simulink model "CoVMD_TrqDesCoord"  (R2016b)
settings: configuration reference "CodeGenConfigSet" (kept outside this file)
values from neighbouring files (symbols this model uses):
  CoVMD_facTrq_C = Calibration.Parameter    [init_CoVMD_TrqDesCoord.m]
  DrvDem_nSetPLo_C = Calibration.Parameter    [init_CoVMD_TrqDesCoord.m]
  VMD_ACCPED = fi(1,State_uint8)    [init_CoVMD_TrqDesCoord.m]
  VMD_CRUISE_CONTROL = fi(2,State_uint8)    [init_CoVMD_TrqDesCoord.m]
  VMD_ENGINE_BRAKE = fi(10,State_uint8)    [init_CoVMD_TrqDesCoord.m]
  VMD_swtVCMActv_C = Calibration.Parameter    [init_CoVMD_TrqDesCoord.m]
undefined symbols (not defined in the file or in its folder): Switch_conv, WESDem_State_conv
libraries: simulink x1
settings Model: Creator=Colin  LastModifiedBy=liutao
settings ConfigSetRef: SourceLocation=Base Workspace

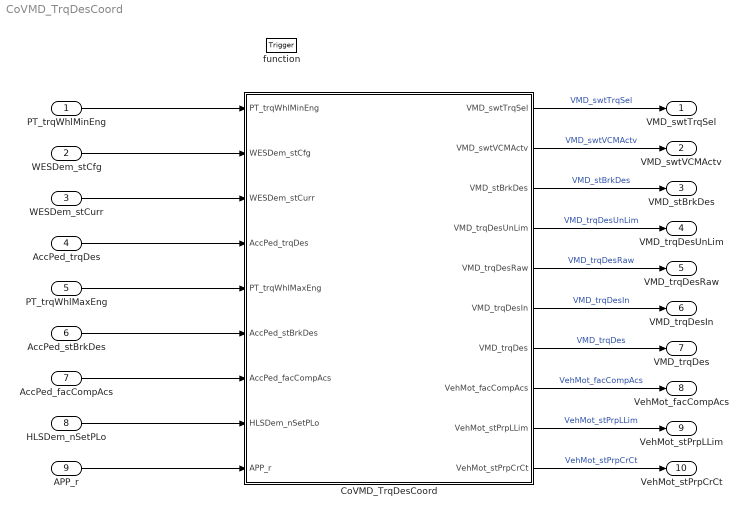
== system CoVMD_TrqDesCoord ==
  PT_trqWhlMinEng : Inport  Tag=Nm  Description=Minimum wheel torque from the engine  OutMin=-3000  OutMax=3000  OutDataTypeStr=Trq_Nm
  WESDem_stCfg : Inport  Description=Configuration of the actual operating mode  Port=2  OutMin=0  OutMax=65535  OutDataTypeStr=State_uint16
  WESDem_stCurr : Inport  Description=Status of the working engine Speed Control  Port=3  OutDataTypeStr=Enum: WESDem_State_conv
  AccPed_trqDes : Inport  Tag=Nm  Description=Driver torque value of propulsion after step limitation  Port=4  OutMin=-3000  OutMax=3000  OutDataTypeStr=Trq_Nm
  PT_trqWhlMaxEng : Inport  Tag=Nm  Description=Maximum wheel torque from the engine  Port=5  OutMin=-3000  OutMax=3000  OutDataTypeStr=Trq_Nm
  AccPed_stBrkDes : Inport  Description=Application parameter for engine brake request  Port=6  OutMin=0  OutMax=255  OutDataTypeStr=State_uint8
  AccPed_facCompAcs : Inport  Description="Factor \"Overrun Ramp\""  Port=7  OutMin=-4  OutMax=3.999  OutDataTypeStr=Fact8192
  HLSDem_nSetPLo : Inport  Tag=rpm  Description=Minimum engine speed of HLSDem  Port=8  OutMin=0  OutMax=6000  OutDataTypeStr=EngSpeed_rpm
  APP_r : Inport  Tag=%  Description=Acceleration pedal sensor 1 value after fault handling  Port=9  OutMin=0  OutMax=100  OutDataTypeStr=Accpedal_rate
  function : TriggerPort  TriggerType=function-call  VariantControl=Variant
  CoVMD_TrqDesCoord : Subsystem
  VMD_swtTrqSel : Outport  Description=Driver demand - Cruise control torque selection switch  OutMin=0  OutMax=255  OutDataTypeStr=State_uint8
  VMD_swtVCMActv : Outport  Description=Application parameter which Indicates whether Vehicle Control Mode(VCM) is enabled or disabled  Port=2  OutDataTypeStr=Enum: Switch_conv
  VMD_stBrkDes : Outport  Description=Application parameter for torque status information  Port=3  OutMin=0  OutMax=65535  OutDataTypeStr=State_uint16
  VMD_trqDesUnLim : Outport  Tag=Nm  Description=Desired torque in front of top speed limitation Nm  Port=4  OutMin=-3000  OutMax=3000  OutDataTypeStr=Trq_Nm
  VMD_trqDesRaw : Outport  Tag=Nm  Description=Raw value of propulsion torque demand.  Port=5  OutMin=-3000  OutMax=3000  OutDataTypeStr=Trq_Nm
  VMD_trqDesIn : Outport  Tag=Nm  Description=Desired Propulsion Torque Nm  Port=6  OutMin=-3000  OutMax=3000  OutDataTypeStr=Trq_Nm
  VMD_trqDes : Outport  Tag=Nm  Description="propulsion  torque after driving assistance coordination"  Port=7  OutMin=-3000  OutMax=3000  OutDataTypeStr=Trq_Nm
  VehMot_facCompAcs : Outport  Description=Compensation factor for loss compensation  Port=8  OutMin=-4  OutMax=3.999  OutDataTypeStr=Fact8192
  VehMot_stPrpLLim : Outport  Description=Status longitudinal limiter controls propulsion torque  Port=9  OutMin=0  OutMax=1  OutDataTypeStr=boolean
  VehMot_stPrpCrCt : Outport  Description=Status cruise control overrides acceleration pedal  Port=10  OutMin=0  OutMax=1  OutDataTypeStr=boolean
  wires:
  PT_trqWhlMinEng/1 -> CoVMD_TrqDesCoord/1(PT_trqWhlMinEng)
  WESDem_stCfg/1 -> CoVMD_TrqDesCoord/2(WESDem_stCfg)
  WESDem_stCurr/1 -> CoVMD_TrqDesCoord/3(WESDem_stCurr)
  AccPed_trqDes/1 -> CoVMD_TrqDesCoord/4(AccPed_trqDes)
  PT_trqWhlMaxEng/1 -> CoVMD_TrqDesCoord/5(PT_trqWhlMaxEng)
  AccPed_stBrkDes/1 -> CoVMD_TrqDesCoord/6(AccPed_stBrkDes)
  AccPed_facCompAcs/1 -> CoVMD_TrqDesCoord/7(AccPed_facCompAcs)
  HLSDem_nSetPLo/1 -> CoVMD_TrqDesCoord/8(HLSDem_nSetPLo)
  APP_r/1 -> CoVMD_TrqDesCoord/9(APP_r)
  CoVMD_TrqDesCoord/1(VMD_swtTrqSel) -> VMD_swtTrqSel/1  "VMD_swtTrqSel"
  CoVMD_TrqDesCoord/2(VMD_swtVCMActv) -> VMD_swtVCMActv/1  "VMD_swtVCMActv"
  CoVMD_TrqDesCoord/3(VMD_stBrkDes) -> VMD_stBrkDes/1  "VMD_stBrkDes"
  CoVMD_TrqDesCoord/4(VMD_trqDesUnLim) -> VMD_trqDesUnLim/1  "VMD_trqDesUnLim"
  CoVMD_TrqDesCoord/5(VMD_trqDesRaw) -> VMD_trqDesRaw/1  "VMD_trqDesRaw"
  CoVMD_TrqDesCoord/6(VMD_trqDesIn) -> VMD_trqDesIn/1  "VMD_trqDesIn"
  CoVMD_TrqDesCoord/7(VMD_trqDes) -> VMD_trqDes/1  "VMD_trqDes"
  CoVMD_TrqDesCoord/8(VehMot_facCompAcs) -> VehMot_facCompAcs/1  "VehMot_facCompAcs"
  CoVMD_TrqDesCoord/9(VehMot_stPrpLLim) -> VehMot_stPrpLLim/1  "VehMot_stPrpLLim"
  CoVMD_TrqDesCoord/10(VehMot_stPrpCrCt) -> VehMot_stPrpCrCt/1  "VehMot_stPrpCrCt"

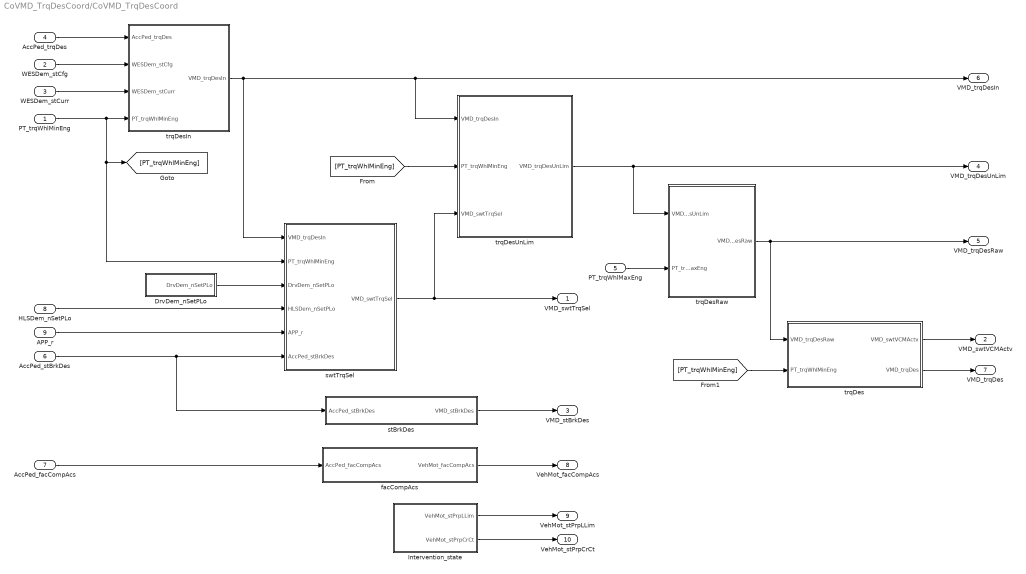
== system CoVMD_TrqDesCoord/CoVMD_TrqDesCoord ==
  PT_trqWhlMinEng : Inport  Tag=Nm  Description=Minimum wheel torque from the engine  OutMin=-3000  OutMax=3000  OutDataTypeStr=Trq_Nm
  WESDem_stCfg : Inport  Description=Configuration of the actual operating mode  Port=2  OutMin=0  OutMax=255
  WESDem_stCurr : Inport  Description=Status of the working engine Speed Control  Port=3  OutDataTypeStr=Enum: WESDem_State_conv
  AccPed_trqDes : Inport  Tag=Nm  Description=driver torque value of propulsion after step limitation  Port=4  OutMin=-3000  OutMax=3000  OutDataTypeStr=Trq_Nm
  PT_trqWhlMaxEng : Inport  Tag=Nm  Description=Maximum wheel torque from the engine  Port=5  OutMin=-3000  OutMax=3000  OutDataTypeStr=Trq_Nm
  AccPed_stBrkDes : Inport  Description=Application parameter for engine brake request  Port=6
  AccPed_facCompAcs : Inport  Description=Compensation factor for loss compensation  Port=7
  HLSDem_nSetPLo : Inport  Tag=rpm  Description=Effective steady-state idle speed  Port=8  OutMin=-12000  OutMax=12000  OutDataTypeStr=EngSpeed_rpm
  APP_r : Inport  Description=Standardized accelerator pedal position  Port=9  OutMin=-400  OutMax=399  OutDataTypeStr=Accpedal_rate
  DrvDem_nSetPLo : Subsystem
  Intervention_state : Subsystem
  facCompAcs : Subsystem
  stBrkDes : Subsystem
  swtTrqSel : Subsystem
  trqDes : Subsystem
  trqDesIn : Subsystem
  trqDesRaw : Subsystem
  trqDesUnLim : Subsystem
  VMD_swtTrqSel : Outport  Description=Driver demand - Cruise control torque selection switch  OutMin=0  OutMax=255  OutDataTypeStr=State_uint8
  VMD_swtVCMActv : Outport  Description=Application parameter which Indicates whether Vehicle Control Mode(VCM) is enabled or disabled  Port=2  OutDataTypeStr=Enum: Switch_conv
  VMD_stBrkDes : Outport  Description=Application parameter for torque status information  Port=3  OutMin=0  OutMax=255
  VMD_trqDesUnLim : Outport  Tag=Nm  Description=Desired torque in front of top speed limitation Nm  Port=4  OutMin=-3000  OutMax=3000  OutDataTypeStr=Trq_Nm
  VMD_trqDesRaw : Outport  Tag=Nm  Description=Raw value of propulsion torque demand.  Port=5  OutMin=-3000  OutMax=3000  OutDataTypeStr=Trq_Nm
  VMD_trqDesIn : Outport  Tag=Nm  Description=Desired Propulsion Torque Nm  Port=6  OutMin=-3000  OutMax=3000  OutDataTypeStr=Trq_Nm
  VMD_trqDes : Outport  Tag=Nm  Description=Propulsion torque after driving assistance coordination  Port=7  OutMin=-3000  OutMax=3000  OutDataTypeStr=Trq_Nm
  VehMot_facCompAcs : Outport  Description=Coordinated factor of accessory compensation  Port=8
  VehMot_stPrpLLim : Outport  Description=Status longitudinal limiter controls propulsion torque  Port=9  OutMin=0  OutMax=1  OutDataTypeStr=boolean
  VehMot_stPrpCrCt : Outport  Description=Status cruise control overrides acceleration pedal  Port=10  OutMin=0  OutMax=1  OutDataTypeStr=boolean
  wires:
  trqDesIn/1(VMD_trqDesIn) -> swtTrqSel/1(VMD_trqDesIn), trqDesUnLim/1(VMD_trqDesIn), VMD_trqDesIn/1
  facCompAcs/1(VehMot_facCompAcs) -> VehMot_facCompAcs/1
  AccPed_facCompAcs/1 -> facCompAcs/1(AccPed_facCompAcs)
  Intervention_state/1(VehMot_stPrpLLim) -> VehMot_stPrpLLim/1
  Intervention_state/2(VehMot_stPrpCrCt) -> VehMot_stPrpCrCt/1
  stBrkDes/1(VMD_stBrkDes) -> VMD_stBrkDes/1
  AccPed_trqDes/1 -> trqDesIn/1(AccPed_trqDes)
  WESDem_stCfg/1 -> trqDesIn/2(WESDem_stCfg)
  PT_trqWhlMinEng/1 -> [PT_trqWhlMinEng], swtTrqSel/2(PT_trqWhlMinEng), trqDesIn/4(PT_trqWhlMinEng)
  WESDem_stCurr/1 -> trqDesIn/3(WESDem_stCurr)
  swtTrqSel/1(VMD_swtTrqSel) -> trqDesUnLim/3(VMD_swtTrqSel), VMD_swtTrqSel/1
  HLSDem_nSetPLo/1 -> swtTrqSel/4(HLSDem_nSetPLo)
  APP_r/1 -> swtTrqSel/5(APP_r)
  AccPed_stBrkDes/1 -> stBrkDes/1(AccPed_stBrkDes), swtTrqSel/6(AccPed_stBrkDes)
  trqDesUnLim/1(VMD_trqDesUnLim) -> VMD_trqDesUnLim/1, trqDesRaw/1(VMD_trqDesUnLim)
  PT_trqWhlMaxEng/1 -> trqDesRaw/2(PT_trqWhlMaxEng)
  trqDesRaw/1(VMD_trqDesRaw) -> VMD_trqDesRaw/1, trqDes/1(VMD_trqDesRaw)
  [PT_trqWhlMinEng] -> trqDesUnLim/2(PT_trqWhlMinEng)
  [PT_trqWhlMinEng] -> trqDes/2(PT_trqWhlMinEng)
  trqDes/2(VMD_trqDes) -> VMD_trqDes/1
  trqDes/1(VMD_swtVCMActv) -> VMD_swtVCMActv/1
  DrvDem_nSetPLo/1(DrvDem_nSetPLo) -> swtTrqSel/3(DrvDem_nSetPLo)

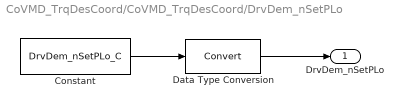
== system CoVMD_TrqDesCoord/CoVMD_TrqDesCoord/DrvDem_nSetPLo ==
  Constant : Constant  Value=DrvDem_nSetPLo_C
  Data Type Conversion : DataTypeConversion
  DrvDem_nSetPLo : Outport
  wires:
  Data Type Conversion/1 -> DrvDem_nSetPLo/1
  Constant/1 -> Data Type Conversion/1

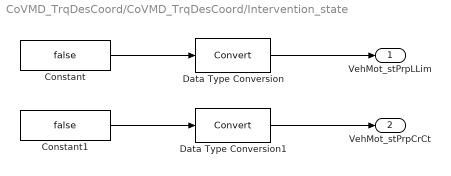
== system CoVMD_TrqDesCoord/CoVMD_TrqDesCoord/Intervention_state ==
  Constant : Constant  Value=false
  Constant1 : Constant  Value=false
  Data Type Conversion : DataTypeConversion
  Data Type Conversion1 : DataTypeConversion
  VehMot_stPrpLLim : Outport  Description=Status longitudinal limiter controls propulsion torque  OutMin=0  OutMax=1  OutDataTypeStr=boolean
  VehMot_stPrpCrCt : Outport  Description=Status cruise control overrides acceleration pedal  Port=2  OutMin=0  OutMax=1  OutDataTypeStr=boolean
  wires:
  Constant/1 -> Data Type Conversion/1
  Constant1/1 -> Data Type Conversion1/1
  Data Type Conversion/1 -> VehMot_stPrpLLim/1
  Data Type Conversion1/1 -> VehMot_stPrpCrCt/1

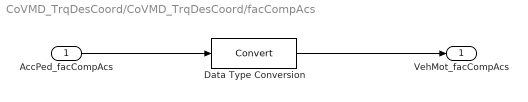
== system CoVMD_TrqDesCoord/CoVMD_TrqDesCoord/facCompAcs ==
  AccPed_facCompAcs : Inport
  Data Type Conversion : DataTypeConversion
  VehMot_facCompAcs : Outport
  wires:
  Data Type Conversion/1 -> VehMot_facCompAcs/1
  AccPed_facCompAcs/1 -> Data Type Conversion/1

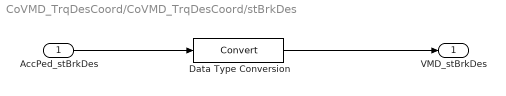
== system CoVMD_TrqDesCoord/CoVMD_TrqDesCoord/stBrkDes ==
  AccPed_stBrkDes : Inport
  Data Type Conversion : DataTypeConversion
  VMD_stBrkDes : Outport
  wires:
  AccPed_stBrkDes/1 -> Data Type Conversion/1
  Data Type Conversion/1 -> VMD_stBrkDes/1

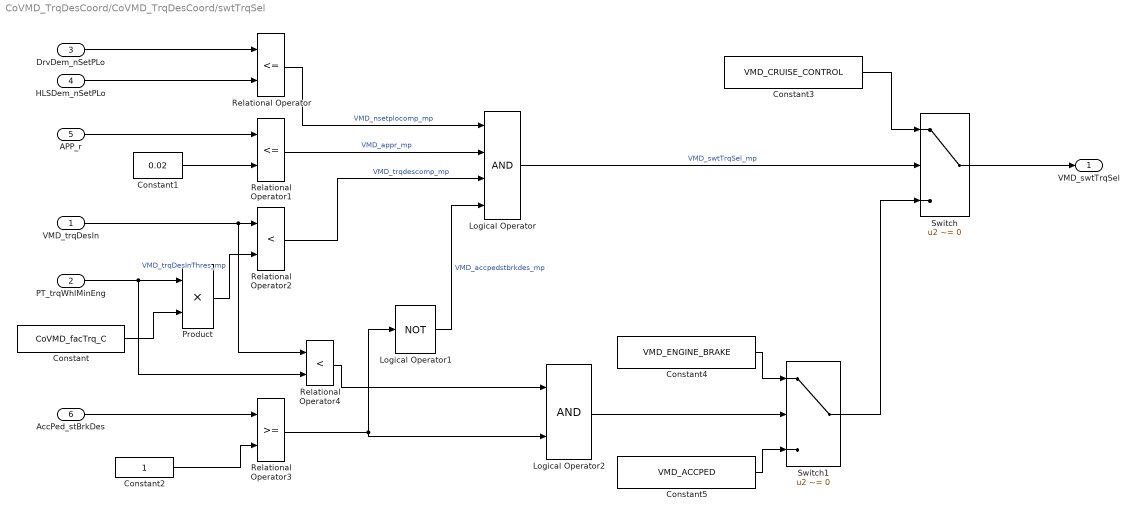
== system CoVMD_TrqDesCoord/CoVMD_TrqDesCoord/swtTrqSel ==
  VMD_trqDesIn : Inport
  PT_trqWhlMinEng : Inport  Tag=Nm  Description=Minimum wheel torque from the engine  Port=2  OutMin=-3000  OutMax=3000  OutDataTypeStr=Trq_Nm
  DrvDem_nSetPLo : Inport  Tag=rpm  Description=Minimal engine speed of DrvDem  Port=3  OutMin=-12000  OutMax=12000  OutDataTypeStr=EngSpeed_rpm
  HLSDem_nSetPLo : Inport  Tag=rpm  Description=Effective steady-state idle speed  Port=4  OutMin=-12000  OutMax=12000  OutDataTypeStr=EngSpeed_rpm
  APP_r : Inport  Description=Standardized accelerator pedal position  Port=5  OutMin=-400  OutMax=399  OutDataTypeStr=Accpedal_rate
  AccPed_stBrkDes : Inport  Description=Application parameter for engine brake request  Port=6
  Constant : Constant  Value=CoVMD_facTrq_C
  Constant1 : Constant  Value=0.02  OutDataTypeStr=Inherit: Inherit via back propagation
  Constant2 : Constant  OutDataTypeStr=Inherit: Inherit via back propagation
  Constant3 : Constant  Value=VMD_CRUISE_CONTROL
  Constant4 : Constant  Value=VMD_ENGINE_BRAKE
  Constant5 : Constant  Value=VMD_ACCPED
  Logical Operator : Logic  Inputs=4  AllPortsSameDT=off  OutDataTypeStr=boolean
  Logical Operator1 : Logic  Operator=NOT  AllPortsSameDT=off  OutDataTypeStr=boolean
  Logical Operator2 : Logic  AllPortsSameDT=off  OutDataTypeStr=boolean
  Product : Product  OutDataTypeStr=Trq_Nm
  Relational Operator : RelationalOperator  Operator=<=  OutDataTypeStr=boolean  RndMeth=Simplest
  Relational Operator1 : RelationalOperator  Operator=<=  OutDataTypeStr=boolean  RndMeth=Simplest  InputSameDT=on
  Relational Operator2 : RelationalOperator  Operator=<  OutDataTypeStr=boolean  RndMeth=Simplest  InputSameDT=on
  Relational Operator3 : RelationalOperator  OutDataTypeStr=boolean  RndMeth=Simplest
  Relational Operator4 : RelationalOperator  Operator=<  OutDataTypeStr=boolean  RndMeth=Simplest
  Switch : Switch  Criteria=u2 ~= 0
  Switch1 : Switch  Criteria=u2 ~= 0
  VMD_swtTrqSel : Outport  Description=Driver demand - Cruise control torque selection switch  OutMin=0  OutMax=255  OutDataTypeStr=State_uint8
  wires:
  DrvDem_nSetPLo/1 -> Relational Operator/1
  HLSDem_nSetPLo/1 -> Relational Operator/2
  Relational Operator/1 -> Logical Operator/1  "VMD_nsetplocomp_mp"
  APP_r/1 -> Relational Operator1/1
  Constant1/1 -> Relational Operator1/2
  Relational Operator1/1 -> Logical Operator/2  "VMD_appr_mp"
  VMD_trqDesIn/1 -> Relational Operator4/1, Relational Operator2/1
  Constant/1 -> Product/2
  PT_trqWhlMinEng/1 -> Relational Operator4/2, Product/1
  Product/1 -> Relational Operator2/2  "VMD_trqDesInThres_mp"
  Relational Operator2/1 -> Logical Operator/3  "VMD_trqdescomp_mp"
  Constant2/1 -> Relational Operator3/2
  AccPed_stBrkDes/1 -> Relational Operator3/1
  Relational Operator3/1 -> Logical Operator2/2, Logical Operator1/1
  Logical Operator1/1 -> Logical Operator/4  "VMD_accpedstbrkdes_mp"
  Logical Operator/1 -> Switch/2  "VMD_swtTrqSel_mp"
  Switch1/1 -> Switch/3
  Constant3/1 -> Switch/1
  Switch/1 -> VMD_swtTrqSel/1
  Logical Operator2/1 -> Switch1/2
  Constant5/1 -> Switch1/3
  Constant4/1 -> Switch1/1
  Relational Operator4/1 -> Logical Operator2/1

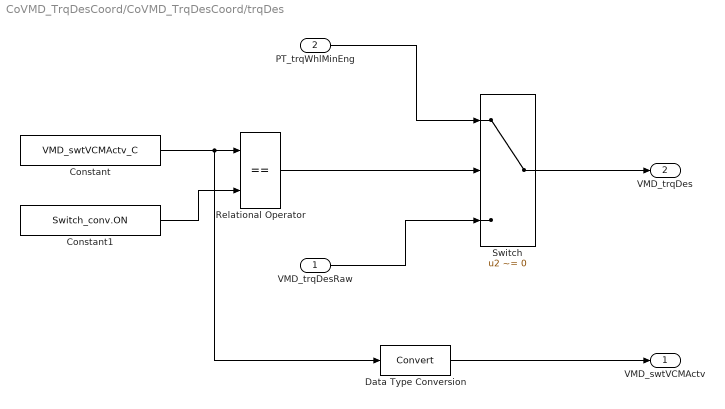
== system CoVMD_TrqDesCoord/CoVMD_TrqDesCoord/trqDes ==
  VMD_trqDesRaw : Inport
  PT_trqWhlMinEng : Inport  Port=2
  Constant : Constant  Value=VMD_swtVCMActv_C
  Constant1 : Constant  Value=Switch_conv.ON
  Data Type Conversion : DataTypeConversion
  Relational Operator : RelationalOperator  Operator===  OutDataTypeStr=boolean  RndMeth=Simplest
  Switch : Switch  Criteria=u2 ~= 0
  VMD_swtVCMActv : Outport
  VMD_trqDes : Outport  Port=2
  wires:
  Constant/1 -> Data Type Conversion/1, Relational Operator/1
  Constant1/1 -> Relational Operator/2
  Relational Operator/1 -> Switch/2
  PT_trqWhlMinEng/1 -> Switch/1
  VMD_trqDesRaw/1 -> Switch/3
  Switch/1 -> VMD_trqDes/1
  Data Type Conversion/1 -> VMD_swtVCMActv/1

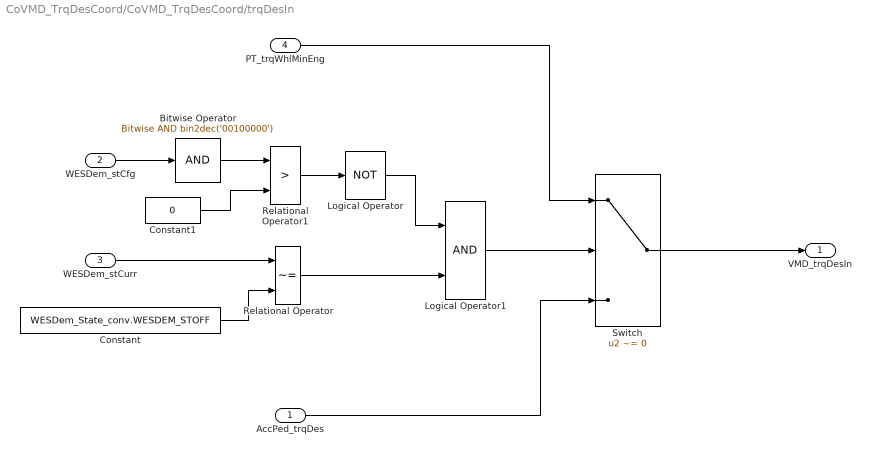
== system CoVMD_TrqDesCoord/CoVMD_TrqDesCoord/trqDesIn ==
  AccPed_trqDes : Inport  Tag=Nm  Description=driver torque value of propulsion after step limitation  OutMin=-3000  OutMax=3000  OutDataTypeStr=Trq_Nm
  WESDem_stCfg : Inport  Description=Configuration of the actual operating mode  Port=2  OutMin=0  OutMax=255
  WESDem_stCurr : Inport  Description=Status of the working engine Speed Control  Port=3  OutDataTypeStr=Enum: WESDem_State_conv
  PT_trqWhlMinEng : Inport  Tag=Nm  Description=Minimum wheel torque from the engine  Port=4  OutMin=-3000  OutMax=3000  OutDataTypeStr=Trq_Nm
  Bitwise Operator : simulink/Logic and Bit Operations/Bitwise Operator  logicop=AND  UseBitMask=on  BitMask=bin2dec('00100000')  BitMaskRealWorld=Stored Integer
  Constant : Constant  Value=WESDem_State_conv.WESDEM_STOFF
  Constant1 : Constant  Value=0  OutDataTypeStr=Inherit: Inherit via back propagation
  Logical Operator : Logic  Operator=NOT  AllPortsSameDT=off  OutDataTypeStr=boolean
  Logical Operator1 : Logic  AllPortsSameDT=off  OutDataTypeStr=boolean
  Relational Operator : RelationalOperator  Operator=~=  OutDataTypeStr=boolean  RndMeth=Simplest
  Relational Operator1 : RelationalOperator  Operator=>  OutDataTypeStr=boolean  RndMeth=Simplest  InputSameDT=on
  Switch : Switch  Criteria=u2 ~= 0
  VMD_trqDesIn : Outport
  wires:
  Constant1/1 -> Relational Operator1/2
  Relational Operator1/1 -> Logical Operator/1
  Constant/1 -> Relational Operator/2
  WESDem_stCurr/1 -> Relational Operator/1
  Relational Operator/1 -> Logical Operator1/2
  Logical Operator/1 -> Logical Operator1/1
  Logical Operator1/1 -> Switch/2
  WESDem_stCfg/1 -> Bitwise Operator/1
  Bitwise Operator/1 -> Relational Operator1/1
  PT_trqWhlMinEng/1 -> Switch/1
  AccPed_trqDes/1 -> Switch/3
  Switch/1 -> VMD_trqDesIn/1

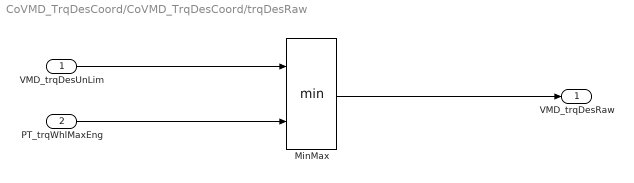
== system CoVMD_TrqDesCoord/CoVMD_TrqDesCoord/trqDesRaw ==
  VMD_trqDesUnLim : Inport
  PT_trqWhlMaxEng : Inport  Port=2
  MinMax : MinMax  Inputs=2
  VMD_trqDesRaw : Outport
  wires:
  MinMax/1 -> VMD_trqDesRaw/1
  VMD_trqDesUnLim/1 -> MinMax/1
  PT_trqWhlMaxEng/1 -> MinMax/2

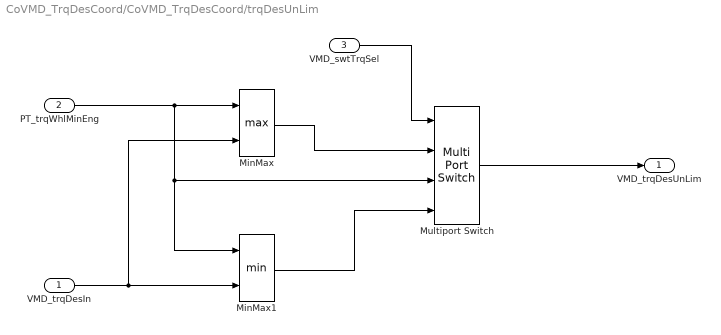
== system CoVMD_TrqDesCoord/CoVMD_TrqDesCoord/trqDesUnLim ==
  VMD_trqDesIn : Inport
  PT_trqWhlMinEng : Inport  Port=2
  VMD_swtTrqSel : Inport  Port=3
  MinMax : MinMax  Function=max  Inputs=2
  MinMax1 : MinMax  Inputs=2
  Multiport Switch : MultiPortSwitch  DataPortOrder=Specify indices  DataPortIndices={1,2,10}
  VMD_trqDesUnLim : Outport  Tag=Nm  Description=Desired torque in front of top speed limitation Nm  OutMin=-3000  OutMax=3000  OutDataTypeStr=Trq_Nm
  wires:
  VMD_swtTrqSel/1 -> Multiport Switch/1
  MinMax/1 -> Multiport Switch/2
  VMD_trqDesIn/1 -> MinMax/2, MinMax1/2
  PT_trqWhlMinEng/1 -> Multiport Switch/3, MinMax1/1, MinMax/1
  MinMax1/1 -> Multiport Switch/4
  Multiport Switch/1 -> VMD_trqDesUnLim/1
